simulink model "gm_hydrophone"  (R2017a)
settings: Solver=FixedStepDiscrete  StartTime=0.0  StopTime=inf  RelTol=1e-3
undefined symbols (not defined in the file or in its folder): coefficients, get
libraries: simulink x6, dspxfrm3 x4, dspmathops x3, dsphdlfiltering x3, dspstat3 x3, dspsnks4 x2, dspsrcs4 x1
settings Model: Creator=jeffr  LastModifiedBy=jeffr
settings SolverCC: AutoInsertRateTranBlk=on
settings DataIOCC: LimitDataPoints=on  SaveOutput=off  SignalLogging=off  SaveTime=off
settings OptimizationCC: BlockReduction=off  ConditionallyExecuteInputs=off  DefaultParameterBehavior=Inlined  LifeSpan=inf
settings DebuggingCC: AlgebraicLoopMsg=error  ArtificialAlgebraicLoopMsg=none  InheritedTsInSrcMsg=none  SingleTaskRateTransMsg=error  AllowSymbolicDim=off  SFUnexpectedBacktrackingDiag=warning  SFNoUnconditionalDefaultTransitionDiag=warning  SFExecutionAtInitializationDiag=none
settings HardwareCC: ProdBitPerPointer=32  ProdBitPerSizeT=32  ProdBitPerPtrDiffT=32  ProdLargestAtomicFloat=None  ProdIntDivRoundTo=Undefined  ProdEndianess=Unspecified  ProdWordSize=32  ProdHWDeviceType=ASIC/FPGA->ASIC/FPGA  ProdEqTarget=off
settings GRTTargetCC: TargetLangStandard=C89/C90 (ANSI)  GeneratePreprocessorConditionals=Disable all
settings ConfigComp: CovMetricSettings=dw  CovHtmlReporting=on  CovSaveCumulativeToWorkspaceVar=on  CovSaveSingleToWorkspaceVar=on  CovExternalEMLEnable=off  CovSFcnEnable=off  DVTestSuiteOptimization=CombinedObjectives (Nonlinear Extended)  DVDetectFloatOverflow=off

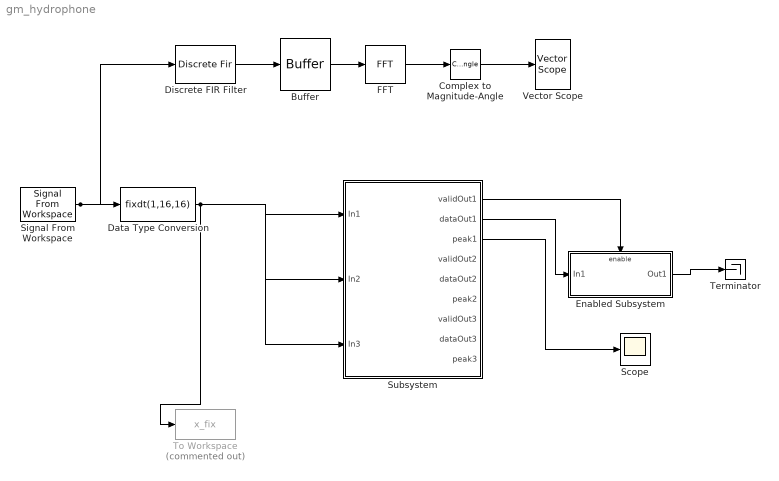
== system gm_hydrophone ==
  Buffer : Buffer  N=1024  OutputFrames=off
  Complex to Magnitude-Angle : ComplexToMagnitudeAngle  Output=Magnitude
  Data Type Conversion : DataTypeConversion  OutDataTypeStr=fixdt(1,16,16)  RndMeth=Round
  Discrete FIR Filter : DiscreteFir  Coefficients=coefficients
  Enabled Subsystem : Subsystem  TreatAsAtomicUnit=on
  FFT : dspxfrm3/FFT  FFTImplementation=Auto  CompMethod=Table lookup  TableOpt=NEW  TableOptActive=Speed  BitRevOrder=off  Normalize=off  InheritFFTLength=on  FFTLength=64  WrapInput=on  roundingMode=Floor  overflowMode=off  firstCoeffDataTypeStr=Inherit: Same word length as input  firstCoeffLastDataTypeStr=Inherit: Same word length as input  outputMin=[]  outputMax=[]
  Scope : Scope
  Signal From Workspace : dspsrcs4/Signal From Workspace  X=x  Ts=2e-6  nsamps=1  OutputAfterFinalValue=Setting to zero  ignoreOrWarnInputAndFrameLengths=off  OutputFrames=off
  Subsystem : Subsystem  TreatAsAtomicUnit=on
  Terminator : Terminator
  To Workspace : ToWorkspace  Commented=on  VariableName=x_fix  SaveFormat=Timeseries  SampleTime=-1
  Vector Scope : dspsnks4/Vector Scope  ScopeProperties=on  Domain=Frequency  HorizSpan=1  DisplayProperties=off  AxisGrid=on  Memory=off  FrameNumber=on  AxisLegend=off  AxisZoom=off  OpenScopeAtSimStart=on  OpenScopeImmediately=off  FigPos=get(0,'defaultfigureposition')  AxisProperties=off  XUnits=Hertz  XRange=[0...Fs/2]  InheritXIncr=on  XIncr=1  XLabel=Time  XLimit=Auto  XMin=0  XMax=1  XStart=0  YUnits=dB  YLabel=Amplitude  LineProperties=off  XAxisParamsVer=6.9
      settings: SourceProductName=DSP System Toolbox  SourceProductBaseCode=DS  YMin=-10  YMax=10
  wires:
  Subsystem/3(peak1) -> Scope/1
  Complex to Magnitude-Angle/1 -> Vector Scope/1
  FFT/1 -> Complex to Magnitude-Angle/1
  Buffer/1 -> FFT/1
  Discrete FIR Filter/1 -> Buffer/1
  Enabled Subsystem/1(Out1) -> Terminator/1
  Subsystem/1(validOut1) -> Enabled Subsystem/Enable
  Subsystem/2(dataOut1) -> Enabled Subsystem/1(In1)
  Signal From Workspace/1 -> Data Type Conversion/1, Discrete FIR Filter/1
  Data Type Conversion/1 -> Subsystem/1(In1), Subsystem/2(In2), Subsystem/3(In3), To Workspace/1

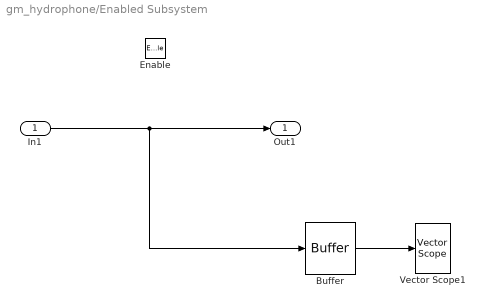
== system gm_hydrophone/Enabled Subsystem ==
  In1 : Inport
  Enable : EnablePort
  Buffer : Buffer  N=1024  OutputFrames=off
  Vector Scope1 : dspsnks4/Vector Scope  ScopeProperties=on  Domain=Frequency  HorizSpan=1  DisplayProperties=off  AxisGrid=on  Memory=off  FrameNumber=on  AxisLegend=off  AxisZoom=off  OpenScopeAtSimStart=on  OpenScopeImmediately=off  FigPos=get(0,'defaultfigureposition')  AxisProperties=off  XUnits=Hertz  XRange=[0...Fs/2]  InheritXIncr=on  XIncr=1  XLabel=Time  XLimit=Auto  XMin=0  XMax=1  XStart=0  YUnits=dB  YLabel=Amplitude  LineProperties=off  XAxisParamsVer=6.9
      settings: SourceProductName=DSP System Toolbox  SourceProductBaseCode=DS  YMin=-10  YMax=10
  Out1 : Outport
  wires:
  Buffer/1 -> Vector Scope1/1
  In1/1 -> Out1/1, Buffer/1

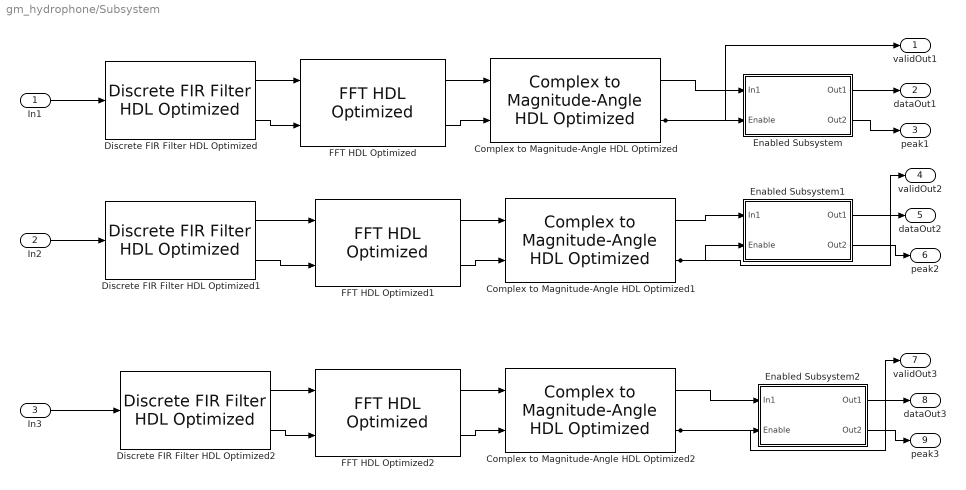
== system gm_hydrophone/Subsystem ==
  In1 : Inport  OutDataTypeStr=fixdt(1, 16, 16)  SampleTime=2e-06
  In2 : Inport  Port=2  OutDataTypeStr=fixdt(1, 16, 16)  SampleTime=2e-06
  In3 : Inport  Port=3  OutDataTypeStr=fixdt(1, 16, 16)  SampleTime=2e-06
  Complex to Magnitude-Angle HDL Optimized : dspmathops/Complex to Magnitude-Angle HDL Optimized  NumIterationsSource=Auto  NumIterations=10  OutputFormat=Magnitude  AngleFormat=Normalized  ScaleOutput=on  SimulateUsing=Code generation
      settings: SourceProductName=DSP System Toolbox  SourceProductBaseCode=DS
  Complex to Magnitude-Angle HDL Optimized1 : dspmathops/Complex to Magnitude-Angle HDL Optimized  NumIterationsSource=Auto  NumIterations=10  OutputFormat=Magnitude  AngleFormat=Normalized  ScaleOutput=on  SimulateUsing=Code generation
      settings: SourceProductName=DSP System Toolbox  SourceProductBaseCode=DS
  Complex to Magnitude-Angle HDL Optimized2 : dspmathops/Complex to Magnitude-Angle HDL Optimized  NumIterationsSource=Auto  NumIterations=10  OutputFormat=Magnitude  AngleFormat=Normalized  ScaleOutput=on  SimulateUsing=Code generation
      settings: SourceProductName=DSP System Toolbox  SourceProductBaseCode=DS
  Discrete FIR Filter HDL Optimized : dsphdlfiltering/Discrete FIR Filter HDL Optimized  Numerator=coefficients  Sharing=off  SharingFactor=2  SimulateUsing=Code generation  roundingMode=Floor  overflowMode=off  CoefficientsDataTypeStr=Inherit: Same word length as input  CoefficientsMin=[]  CoefficientsMax=[]  OutputDataTypeStr=Inherit: Same word length as input  OutputMin=[]  OutputMax=[]  ValidInPort=off  ReadyPort=off
      settings: SourceProductName=DSP System Toolbox  SourceProductBaseCode=DS
  Discrete FIR Filter HDL Optimized1 : dsphdlfiltering/Discrete FIR Filter HDL Optimized  Numerator=coefficients  Sharing=off  SharingFactor=2  SimulateUsing=Code generation  roundingMode=Floor  overflowMode=off  CoefficientsDataTypeStr=Inherit: Same word length as input  CoefficientsMin=[]  CoefficientsMax=[]  OutputDataTypeStr=Inherit: Same word length as input  OutputMin=[]  OutputMax=[]  ValidInPort=off  ReadyPort=off
      settings: SourceProductName=DSP System Toolbox  SourceProductBaseCode=DS
  Discrete FIR Filter HDL Optimized2 : dsphdlfiltering/Discrete FIR Filter HDL Optimized  Numerator=coefficients  Sharing=off  SharingFactor=2  SimulateUsing=Code generation  roundingMode=Floor  overflowMode=off  CoefficientsDataTypeStr=Inherit: Same word length as input  CoefficientsMin=[]  CoefficientsMax=[]  OutputDataTypeStr=Inherit: Same word length as input  OutputMin=[]  OutputMax=[]  ValidInPort=off  ReadyPort=off
      settings: SourceProductName=DSP System Toolbox  SourceProductBaseCode=DS
  Enabled Subsystem : Subsystem
  Enabled Subsystem1 : Subsystem
  Enabled Subsystem2 : Subsystem
  FFT HDL Optimized : dspxfrm3/FFT HDL Optimized  FFTLength=1024  Architecture=Streaming Radix 2^2  ComplexMultiplication=Use 3 multipliers and 5 adders  BitReversedOutput=off  BitReversedInput=off  Normalize=off  SimulateUsing=Code generation  RoundingMethod=Floor  ResetInputPort=off  StartOutputPort=off  EndOutputPort=off
      settings: SourceProductName=DSP System Toolbox  SourceProductBaseCode=DS
  FFT HDL Optimized1 : dspxfrm3/FFT HDL Optimized  FFTLength=1024  Architecture=Streaming Radix 2^2  ComplexMultiplication=Use 3 multipliers and 5 adders  BitReversedOutput=off  BitReversedInput=off  Normalize=off  SimulateUsing=Code generation  RoundingMethod=Floor  ResetInputPort=off  StartOutputPort=off  EndOutputPort=off
      settings: SourceProductName=DSP System Toolbox  SourceProductBaseCode=DS
  FFT HDL Optimized2 : dspxfrm3/FFT HDL Optimized  FFTLength=1024  Architecture=Streaming Radix 2^2  ComplexMultiplication=Use 3 multipliers and 5 adders  BitReversedOutput=off  BitReversedInput=off  Normalize=off  SimulateUsing=Code generation  RoundingMethod=Floor  ResetInputPort=off  StartOutputPort=off  EndOutputPort=off
      settings: SourceProductName=DSP System Toolbox  SourceProductBaseCode=DS
  validOut1 : Outport
  dataOut1 : Outport  Port=2
  peak1 : Outport  Port=3
  validOut2 : Outport  Port=4
  dataOut2 : Outport  Port=5
  peak2 : Outport  Port=6
  validOut3 : Outport  Port=7
  dataOut3 : Outport  Port=8
  peak3 : Outport  Port=9
  wires:
  In1/1 -> Discrete FIR Filter HDL Optimized/1
  In2/1 -> Discrete FIR Filter HDL Optimized1/1
  In3/1 -> Discrete FIR Filter HDL Optimized2/1
  Complex to Magnitude-Angle HDL Optimized/1 -> Enabled Subsystem/1(In1)
  Complex to Magnitude-Angle HDL Optimized/2 -> Enabled Subsystem/2(Enable), validOut1/1
  Complex to Magnitude-Angle HDL Optimized1/1 -> Enabled Subsystem1/1(In1)
  Complex to Magnitude-Angle HDL Optimized1/2 -> validOut2/1, Enabled Subsystem1/2(Enable)
  Complex to Magnitude-Angle HDL Optimized2/1 -> Enabled Subsystem2/1(In1)
  Complex to Magnitude-Angle HDL Optimized2/2 -> validOut3/1, Enabled Subsystem2/2(Enable)
  Discrete FIR Filter HDL Optimized/1 -> FFT HDL Optimized/1
  Discrete FIR Filter HDL Optimized/2 -> FFT HDL Optimized/2
  Discrete FIR Filter HDL Optimized1/1 -> FFT HDL Optimized1/1
  Discrete FIR Filter HDL Optimized1/2 -> FFT HDL Optimized1/2
  Discrete FIR Filter HDL Optimized2/1 -> FFT HDL Optimized2/1
  Discrete FIR Filter HDL Optimized2/2 -> FFT HDL Optimized2/2
  Enabled Subsystem/1(Out1) -> dataOut1/1
  Enabled Subsystem/2(Out2) -> peak1/1
  Enabled Subsystem1/1(Out1) -> dataOut2/1
  Enabled Subsystem1/2(Out2) -> peak2/1
  Enabled Subsystem2/1(Out1) -> dataOut3/1
  Enabled Subsystem2/2(Out2) -> peak3/1
  FFT HDL Optimized/1 -> Complex to Magnitude-Angle HDL Optimized/1
  FFT HDL Optimized/2 -> Complex to Magnitude-Angle HDL Optimized/2
  FFT HDL Optimized1/1 -> Complex to Magnitude-Angle HDL Optimized1/1
  FFT HDL Optimized1/2 -> Complex to Magnitude-Angle HDL Optimized1/2
  FFT HDL Optimized2/1 -> Complex to Magnitude-Angle HDL Optimized2/1
  FFT HDL Optimized2/2 -> Complex to Magnitude-Angle HDL Optimized2/2

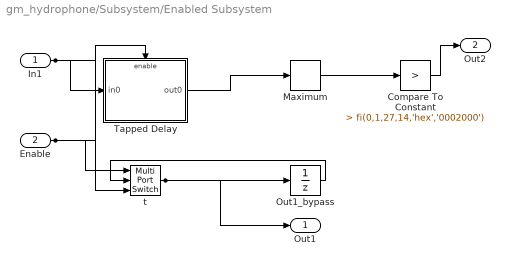
== system gm_hydrophone/Subsystem/Enabled Subsystem ==
  In1 : Inport  SampleTime=2e-06
  Enable : Inport  Port=2  OutDataTypeStr=boolean  SampleTime=2e-06
  Compare To Constant : simulink/Logic and Bit Operations/Compare To Constant  relop=>  const=fi(0,1,27,14,'hex','0002000')  OutDataTypeStr=boolean
  Maximum : dspstat3/Maximum  operation=maximum  fcn=Value  indexBase=One  operateOver=Specified dimension  Dimension=1  InputProcessing=Columns as channels (frame based)  reset=None  roiEnable=off  roiType=Rectangles  roiPortion=Entire ROI  roiOutput=Individual statistics for each ROI  roiFlag=off  roundingMode=Floor  overflowMode=off  accumDataTypeStr=Inherit: Same as product output  accumLastDataTypeStr=Inherit: Same as product output
  Out1_bypass : UnitDelay  SampleTime=2e-06
  Tapped Delay : Subsystem
      settings: MinAlgLoopOccurrences=on
  t : MultiPortSwitch  DataPortOrder=Zero-based contiguous  Inputs=2  zeroidx=on  OutDataTypeStr=fixdt(1, 27, 14)  SampleTime=2e-06
  Out1 : Outport  InitialOutput=0
  Out2 : Outport  Port=2  InitialOutput=0
  wires:
  Enable/1 -> t/1, Tapped Delay/Enable
  In1/1 -> t/3, Tapped Delay/1(in0)
  Compare To Constant/1 -> Out2/1
  Maximum/1 -> Compare To Constant/1
  Tapped Delay/1(out0) -> Maximum/1
  t/1 -> Out1_bypass/1, Out1/1
  Out1_bypass/1 -> t/2

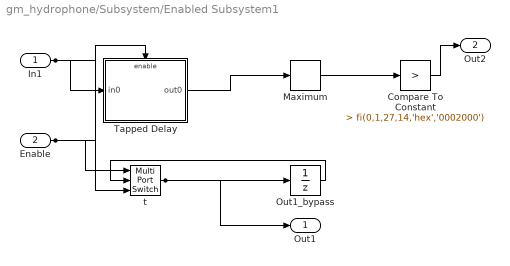
== system gm_hydrophone/Subsystem/Enabled Subsystem1 ==
  In1 : Inport  SampleTime=2e-06
  Enable : Inport  Port=2  OutDataTypeStr=boolean  SampleTime=2e-06
  Compare To Constant : simulink/Logic and Bit Operations/Compare To Constant  relop=>  const=fi(0,1,27,14,'hex','0002000')  OutDataTypeStr=boolean
  Maximum : dspstat3/Maximum  operation=maximum  fcn=Value  indexBase=One  operateOver=Specified dimension  Dimension=1  InputProcessing=Columns as channels (frame based)  reset=None  roiEnable=off  roiType=Rectangles  roiPortion=Entire ROI  roiOutput=Individual statistics for each ROI  roiFlag=off  roundingMode=Floor  overflowMode=off  accumDataTypeStr=Inherit: Same as product output  accumLastDataTypeStr=Inherit: Same as product output
  Out1_bypass : UnitDelay  SampleTime=2e-06
  Tapped Delay : Subsystem
      settings: MinAlgLoopOccurrences=on
  t : MultiPortSwitch  DataPortOrder=Zero-based contiguous  Inputs=2  zeroidx=on  OutDataTypeStr=fixdt(1, 27, 14)  SampleTime=2e-06
  Out1 : Outport  InitialOutput=0
  Out2 : Outport  Port=2  InitialOutput=0
  wires:
  Out1_bypass/1 -> t/2
  t/1 -> Out1/1, Out1_bypass/1
  Tapped Delay/1(out0) -> Maximum/1
  Maximum/1 -> Compare To Constant/1
  Compare To Constant/1 -> Out2/1
  In1/1 -> Tapped Delay/1(in0), t/3
  Enable/1 -> Tapped Delay/Enable, t/1

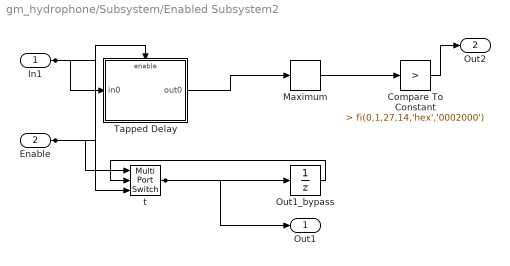
== system gm_hydrophone/Subsystem/Enabled Subsystem2 ==
  In1 : Inport  SampleTime=2e-06
  Enable : Inport  Port=2  OutDataTypeStr=boolean  SampleTime=2e-06
  Compare To Constant : simulink/Logic and Bit Operations/Compare To Constant  relop=>  const=fi(0,1,27,14,'hex','0002000')  OutDataTypeStr=boolean
  Maximum : dspstat3/Maximum  operation=maximum  fcn=Value  indexBase=One  operateOver=Specified dimension  Dimension=1  InputProcessing=Columns as channels (frame based)  reset=None  roiEnable=off  roiType=Rectangles  roiPortion=Entire ROI  roiOutput=Individual statistics for each ROI  roiFlag=off  roundingMode=Floor  overflowMode=off  accumDataTypeStr=Inherit: Same as product output  accumLastDataTypeStr=Inherit: Same as product output
  Out1_bypass : UnitDelay  SampleTime=2e-06
  Tapped Delay : Subsystem
      settings: MinAlgLoopOccurrences=on
  t : MultiPortSwitch  DataPortOrder=Zero-based contiguous  Inputs=2  zeroidx=on  OutDataTypeStr=fixdt(1, 27, 14)  SampleTime=2e-06
  Out1 : Outport  InitialOutput=0
  Out2 : Outport  Port=2  InitialOutput=0
  wires:
  Out1_bypass/1 -> t/2
  t/1 -> Out1/1, Out1_bypass/1
  Tapped Delay/1(out0) -> Maximum/1
  Maximum/1 -> Compare To Constant/1
  Compare To Constant/1 -> Out2/1
  In1/1 -> Tapped Delay/1(in0), t/3
  Enable/1 -> Tapped Delay/Enable, t/1

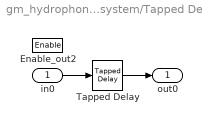
== system gm_hydrophone/Subsystem/Enabled Subsystem/Tapped Delay ==
  in0 : Inport  OutDataTypeStr=fixdt(1, 27, 14)  SampleTime=2e-06
  Enable_out2 : EnablePort  OutDataTypeStr=boolean
  Tapped Delay : simulink/Discrete/Tapped Delay  vinit=0  samptime=-1  NumDelays=hex2num('4090000000000000')  DelayOrder=Oldest  includeCurrent=off
  out0 : Outport  OutDataTypeStr=fixdt(1, 27, 14)  PortDimensions=[1024]  InitialOutput=0
  wires:
  Tapped Delay/1 -> out0/1
  in0/1 -> Tapped Delay/1

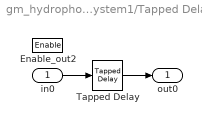
== system gm_hydrophone/Subsystem/Enabled Subsystem1/Tapped Delay ==
  in0 : Inport  OutDataTypeStr=fixdt(1, 27, 14)  SampleTime=2e-06
  Enable_out2 : EnablePort  OutDataTypeStr=boolean
  Tapped Delay : simulink/Discrete/Tapped Delay  vinit=0  samptime=-1  NumDelays=hex2num('4090000000000000')  DelayOrder=Oldest  includeCurrent=off
  out0 : Outport  OutDataTypeStr=fixdt(1, 27, 14)  PortDimensions=[1024]  InitialOutput=0
  wires:
  in0/1 -> Tapped Delay/1
  Tapped Delay/1 -> out0/1

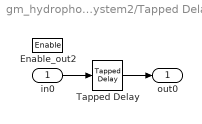
== system gm_hydrophone/Subsystem/Enabled Subsystem2/Tapped Delay ==
  in0 : Inport  OutDataTypeStr=fixdt(1, 27, 14)  SampleTime=2e-06
  Enable_out2 : EnablePort  OutDataTypeStr=boolean
  Tapped Delay : simulink/Discrete/Tapped Delay  vinit=0  samptime=-1  NumDelays=hex2num('4090000000000000')  DelayOrder=Oldest  includeCurrent=off
  out0 : Outport  OutDataTypeStr=fixdt(1, 27, 14)  PortDimensions=[1024]  InitialOutput=0
  wires:
  in0/1 -> Tapped Delay/1
  Tapped Delay/1 -> out0/1
